simulink model "c6_formation"  (R2021b)
settings: Solver=FixedStepDiscrete  StartTime=0.0  StopTime=Inf  FixedStep=sampleTime  RelTol=1e-3  EnableMultiTasking=on
PreLoadFcn:
  | %load emptyMap
  | 
  | % Lidar parameters
  | sensorOffset = [0,0];
  | scanAngles = -pi:pi/6:pi;
  | maxRange = 0.25;
InitFcn:
  | sampleTime = 0.05;
  | nMedianSize=3;
  | 
  | % Robot parameters
  | wheelRadius = 0.0335;
  | robotRadius = 0.116/2;
  | 
  | %角速度坐标
  | ks=1;
  | 
  | % Lidar parameters
  | sensorOffset = [0,0];
  | scanAngles = -pi/3:pi/36:pi/3;
  | maxRange = 0.2;
  | 
  | %车初始位置
  | init_pose_1=[1  1.3  pi/2]';
  | init_pose_2=[0.85 1  pi/2]';
  | init_pose_3=[1.15 1  pi/2]';
  | init_pose_4=[0.7  0.7 pi/2]';
  | init_pose_5=[1  0.7 pi/2]';
  | init_pose_6=[1.3 0.7  pi/2]';
  | 
  | %pp算法性能参数
  | Vd_pp=0.2;
  | Wd_pp=pi;
  | dist_pp=0.2;
  | GoalRadius=0.1;
  | numSector=180;
  | rangeDis=[0.1,maxRange];
  | thresholds=[1/360 1/36];
  | safetyDis=0.2;
  | minimumTurningRadius=0.5*robotRadius;
  | recovery_w=0.05;
undefined symbols (not defined in the file): Angular, DiscIntNeverNeededParam, Linear
libraries: robotlib x24, dspstat3 x18, robotalgslib x6
(part 3 of 4)

== system c6_formation/controller/Car5/ppCar/Adjust Velocities to Avoid Obstacles/Path Following ==
  SteeringDirection : Inport
  V : Inport  Port=2
  AngularVelocity : Inport  Port=3
  Action Port : ActionPort
  Compute Angular Velocity : MATLAB Function  TreatAsAtomicUnit=on
  Constant : Constant  Value=0
  Gain : Gain  Gain=0.2
  MaxAngularVelocity : Constant
  Subtract : Sum  Inputs=+-
  Subtract1 : Sum  Inputs=+-
  dV : Outport  VectorParamsAs1DForOutWhenUnconnected=off
  dW : Outport  Port=2  VectorParamsAs1DForOutWhenUnconnected=off
  wires:
  AngularVelocity/1 -> Subtract/2
  Compute Angular Velocity/1(w) -> Subtract/1
  Subtract/1 -> dW/1
  SteeringDirection/1 -> Compute Angular Velocity/1(steeringDir)
  MaxAngularVelocity/1 -> Compute Angular Velocity/2(wMax)
  Subtract1/1 -> dV/1
  V/1 -> Gain/1
  Constant/1 -> Subtract1/1
  Gain/1 -> Subtract1/2

== system c6_formation/controller/Car5/ppCar/Adjust Velocities to Avoid Obstacles/Recovery ==
  LinearVelocity : Inport
  AngularVelocity : Inport  Port=2
  Action Port : ActionPort
  Constant1 : Constant  Value=-pi/2
  Constant2 : Constant  Value=recovery_w
  Gain : Gain  Gain=-1
  Subtract : Sum  Inputs=+-
  Subtract1 : Sum  Inputs=+-
  dV : Outport  VectorParamsAs1DForOutWhenUnconnected=off
  dW : Outport  Port=2  VectorParamsAs1DForOutWhenUnconnected=off
  wires:
  Subtract/1 -> dW/1
  AngularVelocity/1 -> Subtract/2
  Subtract1/1 -> dV/1
  LinearVelocity/1 -> Gain/1
  Gain/1 -> Subtract1/1
  Constant2/1 -> Subtract1/2
  Constant1/1 -> Subtract/1

== system c6_formation/controller/Car5/ppCar/Compute Velocity and Heading for Path following/Car1 ==
  pose : Inport
  waypoint : Inport  Port=2
  Demux : Demux  Outputs=3
  Demux1 : Demux  Outputs=3
  Ground : Ground
  Kinematicc Controller : Subsystem  mask(Kinematic Controller){kx=2, ky=2, lx=2, ly=2, kw=3, lw=3, Vmax=0.3, Wmax=pi}
      mask prompts: kx "横向偏差增益: kx"; ky "纵向偏差增益: ky"; lx "横向输出饱和: lx"; ly "纵向输出饱和: ly"; kw "离心线速度转角速度增益"; lw "离心线速度转角速度增益"; Vmax "车的限制速度"; Wmax "车的限制角速度"
      mask help: This block implements a controller for differential-drive mobile robots to follow a desired trajectory or to go to a goal point.
      mask Help:
      | This block implements a controller for differential-drive mobile robots to follow a desired trajectory or to go to a goal point.
      | 
      | The trajectory tracking controller is based on the inverse kinematics of the differential-drive robot, whereas only the position [x, y] of the point of interest is considered.
      | It generates references for linear and angular velocities [ud, wd] based on the robot's actual pose [x, y, psi] deseired position [xd, yd] and desired speed [dxd, dyd].
      | 
      | The constant "a" represents the distance of the point of interest [x, y] to the center of the line that connects the traction wheels.
      | 
      | <b>Parameters:</b>
      | 
      | kx > 0 and ky > 0: controller gains;
      | lx > 0 and ly > 0: saturation constants.
      | 
      | 
      | <b>Inputs:</b>
      | 
      | psi: actual robot orientation [rad] (psi=0 means the robot orientation is the same as the x axis);
      | x: actual robot position [m] in x axis;
      | xd: desired robot position [m] in x axis;
      | dxd: desired robot speed [m/s] in x axis;
      | y: actual robot position [m] in y axis;
      | yd: desired robot position [m] in y axis;
      | dyd: desired robot speed [m/s] in y axis;
      | 
      | <b>Outputs:</b>
      | 
      | ud: reference for linear velocity [m/s]
      | wd: reference for angular velocity [rad/s]
      | 
      | 
      | <b>Notes:</b>
      | 
      | If the deseired position [xd, yd] is constant and the desired speed [dxd, dyd] is zero, the controller works as a position controller: it drives the robot to a goal position [xd, yd].
      | 
      | ------
      | For detailed information on the system, please refer to the following papers and thesis:
      | 
      | [1] MARTINS, F. N., Celeste, W. C., Carelli, R., Sarcinelli-Filho, M. and
      | Bastos-Filho, T. F. An Adaptive Dynamic Controller for Autonomous Mobile Robot
      | Trajectory Tracking. Control Engineering Practice, v. 16, p. 1354–1363, 2008.
      | doi: 10.1016/j.conengprac.2008.03.004
      | 
      | [2] MARTINS, F. N., Carelli, R., Sarcinelli-Filho, M. and Bastos-Filho, T. F.
      | Dynamic Modeling and Adaptive Dynamic Compensation for Unicycle-Like
      | Mobile Robots. 14th International Conference on Advanced Robotics -
      | ICAR 2009, Germany, June, 22-26, 2009.
      | 
      | [3] Thesis: "Modelagem e Compensacao da Dinamica de Robos Moveis e sua
      | Aplicacao em Controle de Formacao". Felipe Nascimento Martins. Tese de
      | Doutorado em Engenharia Eletrica - Automacao. UFES, 2009.
      | 
      | ---
      | Based on a prior work by Felipe Nascimento Martins and Wanderley Cardoso Celeste
      | UFES - Federal University of Espirito Santo, BRAZIL
      | 2006--2008
      | 
      | Author: Felipe Nascimento Martins
      | Federal Institute of Education, Science and Technology of Espirito Santo - IFES
      | NERA - Núcleo de Estudos em Robótica e Automação
      | http://nera.sr.ifes.edu.br
      | MAY/2013
      | Blog sobre robótica: www.nossosrobos.blogspot.com
  V : Outport
  W : Outport  Port=2
  targetdir : Outport  Port=3
  wires:
  Ground/1 -> Kinematicc Controller/7(dxd), Kinematicc Controller/8(dyd)
  Demux1/2 -> Kinematicc Controller/5(yd)
  Kinematicc Controller/1(ud) -> V/1  "速度指令"
  Demux/2 -> Kinematicc Controller/2(y)
  pose/1 -> Demux/1
  Demux/3 -> Kinematicc Controller/3(psi)
  Demux/1 -> Kinematicc Controller/1(x)
  Kinematicc Controller/2(wd) -> W/1  "角速度指令"
  Demux1/1 -> Kinematicc Controller/4(xd)
  waypoint/1 -> Demux1/1
  Demux1/3 -> Kinematicc Controller/6(psid)
  Kinematicc Controller/3(targetdir) -> targetdir/1

== system c6_formation/controller/Car6/ppCar/Adjust Velocities to Avoid Obstacles/Path Following ==
  SteeringDirection : Inport
  V : Inport  Port=2
  AngularVelocity : Inport  Port=3
  Action Port : ActionPort
  Compute Angular Velocity : MATLAB Function  TreatAsAtomicUnit=on
  Constant : Constant  Value=0
  Gain : Gain  Gain=0.2
  MaxAngularVelocity : Constant
  Subtract : Sum  Inputs=+-
  Subtract1 : Sum  Inputs=+-
  dV : Outport  VectorParamsAs1DForOutWhenUnconnected=off
  dW : Outport  Port=2  VectorParamsAs1DForOutWhenUnconnected=off
  wires:
  Gain/1 -> Subtract1/2
  Constant/1 -> Subtract1/1
  V/1 -> Gain/1
  Subtract1/1 -> dV/1
  MaxAngularVelocity/1 -> Compute Angular Velocity/2(wMax)
  SteeringDirection/1 -> Compute Angular Velocity/1(steeringDir)
  Subtract/1 -> dW/1
  Compute Angular Velocity/1(w) -> Subtract/1
  AngularVelocity/1 -> Subtract/2

== system c6_formation/controller/Car6/ppCar/Adjust Velocities to Avoid Obstacles/Recovery ==
  LinearVelocity : Inport
  AngularVelocity : Inport  Port=2
  Action Port : ActionPort
  Constant1 : Constant  Value=-pi/2
  Constant2 : Constant  Value=recovery_w
  Gain : Gain  Gain=-1
  Subtract : Sum  Inputs=+-
  Subtract1 : Sum  Inputs=+-
  dV : Outport  VectorParamsAs1DForOutWhenUnconnected=off
  dW : Outport  Port=2  VectorParamsAs1DForOutWhenUnconnected=off
  wires:
  Constant1/1 -> Subtract/1
  Constant2/1 -> Subtract1/2
  Gain/1 -> Subtract1/1
  LinearVelocity/1 -> Gain/1
  Subtract1/1 -> dV/1
  AngularVelocity/1 -> Subtract/2
  Subtract/1 -> dW/1

== system c6_formation/controller/Car6/ppCar/Compute Velocity and Heading for Path following/Car1 ==
  pose : Inport
  waypoint : Inport  Port=2
  Demux : Demux  Outputs=3
  Demux1 : Demux  Outputs=3
  Ground : Ground
  Kinematicc Controller : Subsystem  mask(Kinematic Controller){kx=2, ky=2, lx=2, ly=2, kw=3, lw=3, Vmax=0.3, Wmax=pi}
      mask prompts: kx "横向偏差增益: kx"; ky "纵向偏差增益: ky"; lx "横向输出饱和: lx"; ly "纵向输出饱和: ly"; kw "离心线速度转角速度增益"; lw "离心线速度转角速度增益"; Vmax "车的限制速度"; Wmax "车的限制角速度"
      mask help: This block implements a controller for differential-drive mobile robots to follow a desired trajectory or to go to a goal point.
      mask Help:
      | This block implements a controller for differential-drive mobile robots to follow a desired trajectory or to go to a goal point.
      | 
      | The trajectory tracking controller is based on the inverse kinematics of the differential-drive robot, whereas only the position [x, y] of the point of interest is considered.
      | It generates references for linear and angular velocities [ud, wd] based on the robot's actual pose [x, y, psi] deseired position [xd, yd] and desired speed [dxd, dyd].
      | 
      | The constant "a" represents the distance of the point of interest [x, y] to the center of the line that connects the traction wheels.
      | 
      | <b>Parameters:</b>
      | 
      | kx > 0 and ky > 0: controller gains;
      | lx > 0 and ly > 0: saturation constants.
      | 
      | 
      | <b>Inputs:</b>
      | 
      | psi: actual robot orientation [rad] (psi=0 means the robot orientation is the same as the x axis);
      | x: actual robot position [m] in x axis;
      | xd: desired robot position [m] in x axis;
      | dxd: desired robot speed [m/s] in x axis;
      | y: actual robot position [m] in y axis;
      | yd: desired robot position [m] in y axis;
      | dyd: desired robot speed [m/s] in y axis;
      | 
      | <b>Outputs:</b>
      | 
      | ud: reference for linear velocity [m/s]
      | wd: reference for angular velocity [rad/s]
      | 
      | 
      | <b>Notes:</b>
      | 
      | If the deseired position [xd, yd] is constant and the desired speed [dxd, dyd] is zero, the controller works as a position controller: it drives the robot to a goal position [xd, yd].
      | 
      | ------
      | For detailed information on the system, please refer to the following papers and thesis:
      | 
      | [1] MARTINS, F. N., Celeste, W. C., Carelli, R., Sarcinelli-Filho, M. and
      | Bastos-Filho, T. F. An Adaptive Dynamic Controller for Autonomous Mobile Robot
      | Trajectory Tracking. Control Engineering Practice, v. 16, p. 1354–1363, 2008.
      | doi: 10.1016/j.conengprac.2008.03.004
      | 
      | [2] MARTINS, F. N., Carelli, R., Sarcinelli-Filho, M. and Bastos-Filho, T. F.
      | Dynamic Modeling and Adaptive Dynamic Compensation for Unicycle-Like
      | Mobile Robots. 14th International Conference on Advanced Robotics -
      | ICAR 2009, Germany, June, 22-26, 2009.
      | 
      | [3] Thesis: "Modelagem e Compensacao da Dinamica de Robos Moveis e sua
      | Aplicacao em Controle de Formacao". Felipe Nascimento Martins. Tese de
      | Doutorado em Engenharia Eletrica - Automacao. UFES, 2009.
      | 
      | ---
      | Based on a prior work by Felipe Nascimento Martins and Wanderley Cardoso Celeste
      | UFES - Federal University of Espirito Santo, BRAZIL
      | 2006--2008
      | 
      | Author: Felipe Nascimento Martins
      | Federal Institute of Education, Science and Technology of Espirito Santo - IFES
      | NERA - Núcleo de Estudos em Robótica e Automação
      | http://nera.sr.ifes.edu.br
      | MAY/2013
      | Blog sobre robótica: www.nossosrobos.blogspot.com
  V : Outport
  W : Outport  Port=2
  targetdir : Outport  Port=3
  wires:
  Kinematicc Controller/3(targetdir) -> targetdir/1
  Demux1/3 -> Kinematicc Controller/6(psid)
  waypoint/1 -> Demux1/1
  Demux1/1 -> Kinematicc Controller/4(xd)
  Kinematicc Controller/2(wd) -> W/1  "角速度指令"
  Demux/1 -> Kinematicc Controller/1(x)
  Demux/3 -> Kinematicc Controller/3(psi)
  pose/1 -> Demux/1
  Demux/2 -> Kinematicc Controller/2(y)
  Kinematicc Controller/1(ud) -> V/1  "速度指令"
  Demux1/2 -> Kinematicc Controller/5(yd)
  Ground/1 -> Kinematicc Controller/8(dyd), Kinematicc Controller/7(dxd)

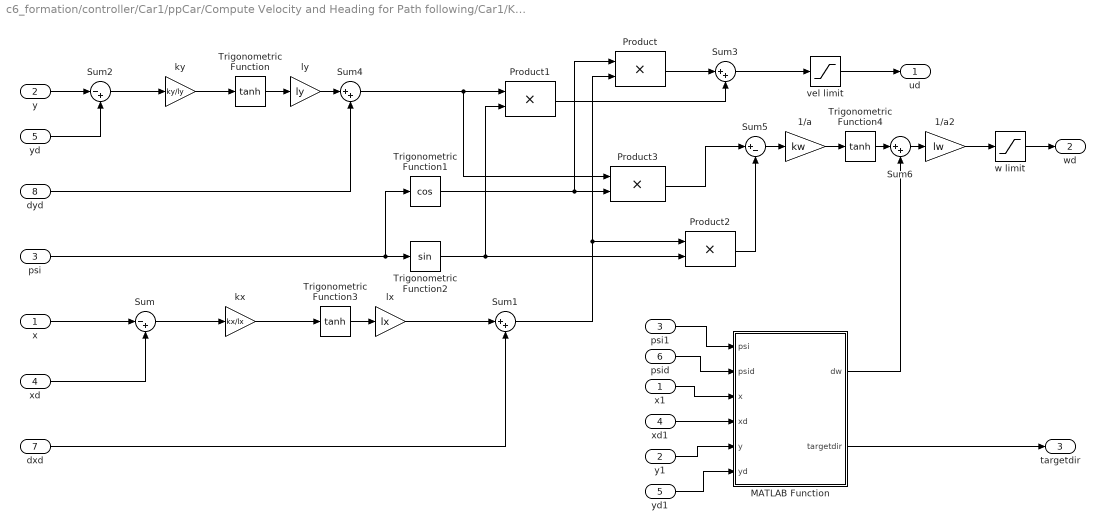
== system c6_formation/controller/Car1/ppCar/Compute Velocity and Heading for Path following/Car1/Kinematicc Controller ==
  x : Inport
  y : Inport  Port=2
  psi : Inport  Port=3
  xd : Inport  Port=4
  yd : Inport  Port=5
  psid : Inport  Port=6
  dxd : Inport  Port=7
  dyd : Inport  Port=8
  1/a : Gain  Gain=kw  SaturateOnIntegerOverflow=on  OutDataTypeStr=Inherit: Same as input  ParamDataTypeStr=Inherit: Same as input
  1/a2 : Gain  Gain=lw  SaturateOnIntegerOverflow=on  OutDataTypeStr=Inherit: Same as input  ParamDataTypeStr=Inherit: Same as input
  MATLAB Function : MATLAB Function  TreatAsAtomicUnit=on
  Product{,1..3} (4 alike) : Product  SaturateOnIntegerOverflow=on  OutDataTypeStr=Inherit: Same as first input
  Sum : Sum  Inputs=|-+  SaturateOnIntegerOverflow=on
  Sum{1,3..4,6} (4 alike) : Sum  Inputs=|++  SaturateOnIntegerOverflow=on
  Sum2 : Sum  Inputs=|-+  SaturateOnIntegerOverflow=on
  Sum5 : Sum  Inputs=|+-  SaturateOnIntegerOverflow=on
  Trigonometric Function : Trigonometry  Operator=tanh
  Trigonometric Function1 : Trigonometry  Operator=cos
  Trigonometric Function2 : Trigonometry
  Trigonometric Function3 : Trigonometry  Operator=tanh
  Trigonometric Function4 : Trigonometry  Operator=tanh
  kx : Gain  Gain=kx/lx  SaturateOnIntegerOverflow=on  OutDataTypeStr=Inherit: Same as input  ParamDataTypeStr=Inherit: Same as input
  ky : Gain  Gain=ky/ly  SaturateOnIntegerOverflow=on  OutDataTypeStr=Inherit: Same as input  ParamDataTypeStr=Inherit: Same as input
  lx : Gain  Gain=lx  SaturateOnIntegerOverflow=on  OutDataTypeStr=Inherit: Same as input  ParamDataTypeStr=Inherit: Same as input
  ly : Gain  Gain=ly  SaturateOnIntegerOverflow=on  OutDataTypeStr=Inherit: Same as input  ParamDataTypeStr=Inherit: Same as input
  psi1 : InportShadow  Port=3
  vel limit : Saturate  UpperLimit=Vmax  LowerLimit=-0.4*Vmax
  w limit : Saturate  UpperLimit=Wmax  LowerLimit=-Wmax
  x1 : InportShadow
  xd1 : InportShadow  Port=4
  y1 : InportShadow  Port=2
  yd1 : InportShadow  Port=5
  ud : Outport
  wd : Outport  Port=2
  targetdir : Outport  Port=3
  wires:
  kx/1 -> Trigonometric Function3/1
  ky/1 -> Trigonometric Function/1
  Trigonometric Function1/1 -> Product3/2, Product/1
  Sum/1 -> kx/1
  y/1 -> Sum2/1
  Sum4/1 -> Product1/1, Product3/1
  Trigonometric Function2/1 -> Product2/2, Product1/2
  Sum3/1 -> vel limit/1
  dxd/1 -> Sum1/2
  dyd/1 -> Sum4/2
  ly/1 -> Sum4/1
  Trigonometric Function/1 -> ly/1
  lx/1 -> Sum1/1
  Trigonometric Function3/1 -> lx/1
  yd/1 -> Sum2/2
  xd/1 -> Sum/2
  x/1 -> Sum/1
  psi/1 -> Trigonometric Function2/1, Trigonometric Function1/1
  Sum1/1 -> Product2/1, Product/2
  Sum2/1 -> ky/1
  Product/1 -> Sum3/1
  Product1/1 -> Sum3/2
  Product3/1 -> Sum5/1
  Product2/1 -> Sum5/2
  Sum5/1 -> 1/a/1
  Trigonometric Function4/1 -> Sum6/1
  1/a/1 -> Trigonometric Function4/1
  vel limit/1 -> ud/1
  w limit/1 -> wd/1
  1/a2/1 -> w limit/1
  Sum6/1 -> 1/a2/1
  psid/1 -> MATLAB Function/2(psid)
  psi1/1 -> MATLAB Function/1(psi)
  x1/1 -> MATLAB Function/3(x)
  xd1/1 -> MATLAB Function/4(xd)
  y1/1 -> MATLAB Function/5(y)
  yd1/1 -> MATLAB Function/6(yd)
  MATLAB Function/1(dw) -> Sum6/2
  MATLAB Function/2(targetdir) -> targetdir/1

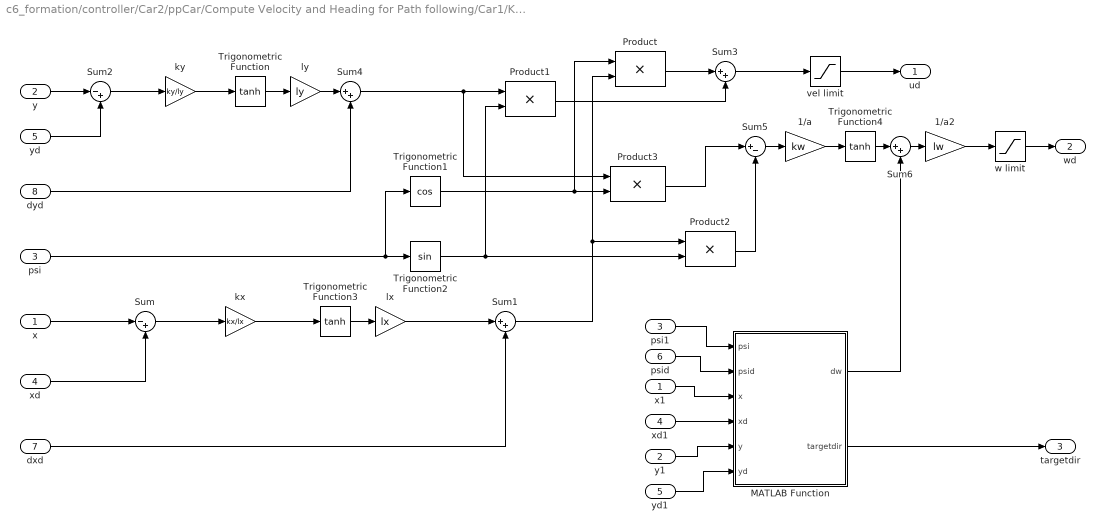
== system c6_formation/controller/Car2/ppCar/Compute Velocity and Heading for Path following/Car1/Kinematicc Controller ==
  x : Inport
  y : Inport  Port=2
  psi : Inport  Port=3
  xd : Inport  Port=4
  yd : Inport  Port=5
  psid : Inport  Port=6
  dxd : Inport  Port=7
  dyd : Inport  Port=8
  1/a : Gain  Gain=kw  SaturateOnIntegerOverflow=on  OutDataTypeStr=Inherit: Same as input  ParamDataTypeStr=Inherit: Same as input
  1/a2 : Gain  Gain=lw  SaturateOnIntegerOverflow=on  OutDataTypeStr=Inherit: Same as input  ParamDataTypeStr=Inherit: Same as input
  MATLAB Function : MATLAB Function  TreatAsAtomicUnit=on
  Product{,1..3} (4 alike) : Product  SaturateOnIntegerOverflow=on  OutDataTypeStr=Inherit: Same as first input
  Sum : Sum  Inputs=|-+  SaturateOnIntegerOverflow=on
  Sum{1,3..4,6} (4 alike) : Sum  Inputs=|++  SaturateOnIntegerOverflow=on
  Sum2 : Sum  Inputs=|-+  SaturateOnIntegerOverflow=on
  Sum5 : Sum  Inputs=|+-  SaturateOnIntegerOverflow=on
  Trigonometric Function : Trigonometry  Operator=tanh
  Trigonometric Function1 : Trigonometry  Operator=cos
  Trigonometric Function2 : Trigonometry
  Trigonometric Function3 : Trigonometry  Operator=tanh
  Trigonometric Function4 : Trigonometry  Operator=tanh
  kx : Gain  Gain=kx/lx  SaturateOnIntegerOverflow=on  OutDataTypeStr=Inherit: Same as input  ParamDataTypeStr=Inherit: Same as input
  ky : Gain  Gain=ky/ly  SaturateOnIntegerOverflow=on  OutDataTypeStr=Inherit: Same as input  ParamDataTypeStr=Inherit: Same as input
  lx : Gain  Gain=lx  SaturateOnIntegerOverflow=on  OutDataTypeStr=Inherit: Same as input  ParamDataTypeStr=Inherit: Same as input
  ly : Gain  Gain=ly  SaturateOnIntegerOverflow=on  OutDataTypeStr=Inherit: Same as input  ParamDataTypeStr=Inherit: Same as input
  psi1 : InportShadow  Port=3
  vel limit : Saturate  UpperLimit=Vmax  LowerLimit=-0.4*Vmax
  w limit : Saturate  UpperLimit=Wmax  LowerLimit=-Wmax
  x1 : InportShadow
  xd1 : InportShadow  Port=4
  y1 : InportShadow  Port=2
  yd1 : InportShadow  Port=5
  ud : Outport
  wd : Outport  Port=2
  targetdir : Outport  Port=3
  wires:
  MATLAB Function/2(targetdir) -> targetdir/1
  MATLAB Function/1(dw) -> Sum6/2
  yd1/1 -> MATLAB Function/6(yd)
  y1/1 -> MATLAB Function/5(y)
  xd1/1 -> MATLAB Function/4(xd)
  x1/1 -> MATLAB Function/3(x)
  psi1/1 -> MATLAB Function/1(psi)
  psid/1 -> MATLAB Function/2(psid)
  Sum6/1 -> 1/a2/1
  1/a2/1 -> w limit/1
  w limit/1 -> wd/1
  vel limit/1 -> ud/1
  1/a/1 -> Trigonometric Function4/1
  Trigonometric Function4/1 -> Sum6/1
  Sum5/1 -> 1/a/1
  Product2/1 -> Sum5/2
  Product3/1 -> Sum5/1
  Product1/1 -> Sum3/2
  Product/1 -> Sum3/1
  Sum2/1 -> ky/1
  Sum1/1 -> Product/2, Product2/1
  psi/1 -> Trigonometric Function1/1, Trigonometric Function2/1
  x/1 -> Sum/1
  xd/1 -> Sum/2
  yd/1 -> Sum2/2
  Trigonometric Function3/1 -> lx/1
  lx/1 -> Sum1/1
  Trigonometric Function/1 -> ly/1
  ly/1 -> Sum4/1
  dyd/1 -> Sum4/2
  dxd/1 -> Sum1/2
  Sum3/1 -> vel limit/1
  Trigonometric Function2/1 -> Product1/2, Product2/2
  Sum4/1 -> Product3/1, Product1/1
  y/1 -> Sum2/1
  Sum/1 -> kx/1
  Trigonometric Function1/1 -> Product/1, Product3/2
  ky/1 -> Trigonometric Function/1
  kx/1 -> Trigonometric Function3/1

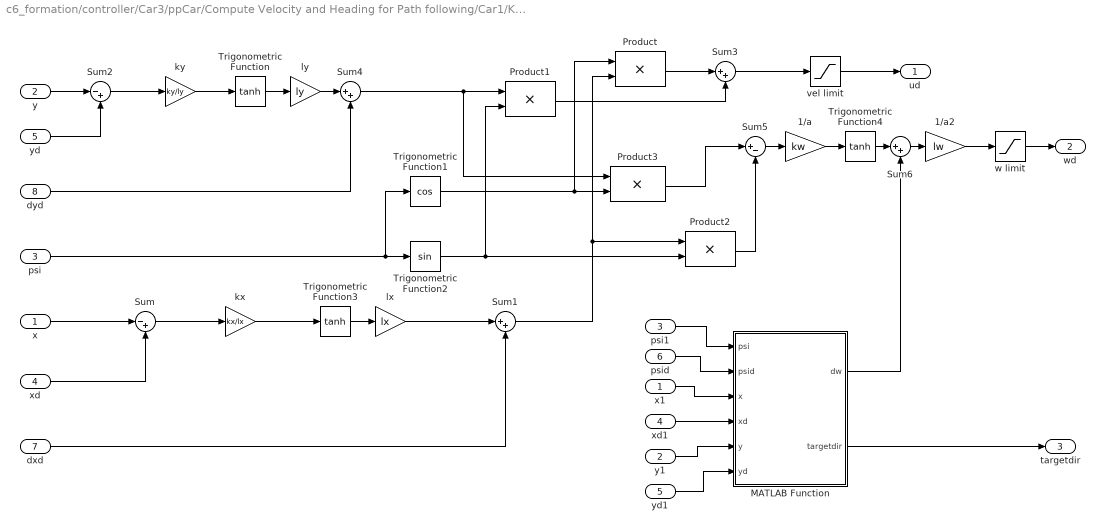
== system c6_formation/controller/Car3/ppCar/Compute Velocity and Heading for Path following/Car1/Kinematicc Controller ==
  x : Inport
  y : Inport  Port=2
  psi : Inport  Port=3
  xd : Inport  Port=4
  yd : Inport  Port=5
  psid : Inport  Port=6
  dxd : Inport  Port=7
  dyd : Inport  Port=8
  1/a : Gain  Gain=kw  SaturateOnIntegerOverflow=on  OutDataTypeStr=Inherit: Same as input  ParamDataTypeStr=Inherit: Same as input
  1/a2 : Gain  Gain=lw  SaturateOnIntegerOverflow=on  OutDataTypeStr=Inherit: Same as input  ParamDataTypeStr=Inherit: Same as input
  MATLAB Function : MATLAB Function  TreatAsAtomicUnit=on
  Product{,1..3} (4 alike) : Product  SaturateOnIntegerOverflow=on  OutDataTypeStr=Inherit: Same as first input
  Sum : Sum  Inputs=|-+  SaturateOnIntegerOverflow=on
  Sum{1,3..4,6} (4 alike) : Sum  Inputs=|++  SaturateOnIntegerOverflow=on
  Sum2 : Sum  Inputs=|-+  SaturateOnIntegerOverflow=on
  Sum5 : Sum  Inputs=|+-  SaturateOnIntegerOverflow=on
  Trigonometric Function : Trigonometry  Operator=tanh
  Trigonometric Function1 : Trigonometry  Operator=cos
  Trigonometric Function2 : Trigonometry
  Trigonometric Function3 : Trigonometry  Operator=tanh
  Trigonometric Function4 : Trigonometry  Operator=tanh
  kx : Gain  Gain=kx/lx  SaturateOnIntegerOverflow=on  OutDataTypeStr=Inherit: Same as input  ParamDataTypeStr=Inherit: Same as input
  ky : Gain  Gain=ky/ly  SaturateOnIntegerOverflow=on  OutDataTypeStr=Inherit: Same as input  ParamDataTypeStr=Inherit: Same as input
  lx : Gain  Gain=lx  SaturateOnIntegerOverflow=on  OutDataTypeStr=Inherit: Same as input  ParamDataTypeStr=Inherit: Same as input
  ly : Gain  Gain=ly  SaturateOnIntegerOverflow=on  OutDataTypeStr=Inherit: Same as input  ParamDataTypeStr=Inherit: Same as input
  psi1 : InportShadow  Port=3
  vel limit : Saturate  UpperLimit=Vmax  LowerLimit=-0.4*Vmax
  w limit : Saturate  UpperLimit=Wmax  LowerLimit=-Wmax
  x1 : InportShadow
  xd1 : InportShadow  Port=4
  y1 : InportShadow  Port=2
  yd1 : InportShadow  Port=5
  ud : Outport
  wd : Outport  Port=2
  targetdir : Outport  Port=3
  wires:
  kx/1 -> Trigonometric Function3/1
  ky/1 -> Trigonometric Function/1
  Trigonometric Function1/1 -> Product3/2, Product/1
  Sum/1 -> kx/1
  y/1 -> Sum2/1
  Sum4/1 -> Product1/1, Product3/1
  Trigonometric Function2/1 -> Product2/2, Product1/2
  Sum3/1 -> vel limit/1
  dxd/1 -> Sum1/2
  dyd/1 -> Sum4/2
  ly/1 -> Sum4/1
  Trigonometric Function/1 -> ly/1
  lx/1 -> Sum1/1
  Trigonometric Function3/1 -> lx/1
  yd/1 -> Sum2/2
  xd/1 -> Sum/2
  x/1 -> Sum/1
  psi/1 -> Trigonometric Function2/1, Trigonometric Function1/1
  Sum1/1 -> Product2/1, Product/2
  Sum2/1 -> ky/1
  Product/1 -> Sum3/1
  Product1/1 -> Sum3/2
  Product3/1 -> Sum5/1
  Product2/1 -> Sum5/2
  Sum5/1 -> 1/a/1
  Trigonometric Function4/1 -> Sum6/1
  1/a/1 -> Trigonometric Function4/1
  vel limit/1 -> ud/1
  w limit/1 -> wd/1
  1/a2/1 -> w limit/1
  Sum6/1 -> 1/a2/1
  psid/1 -> MATLAB Function/2(psid)
  psi1/1 -> MATLAB Function/1(psi)
  x1/1 -> MATLAB Function/3(x)
  xd1/1 -> MATLAB Function/4(xd)
  y1/1 -> MATLAB Function/5(y)
  yd1/1 -> MATLAB Function/6(yd)
  MATLAB Function/1(dw) -> Sum6/2
  MATLAB Function/2(targetdir) -> targetdir/1

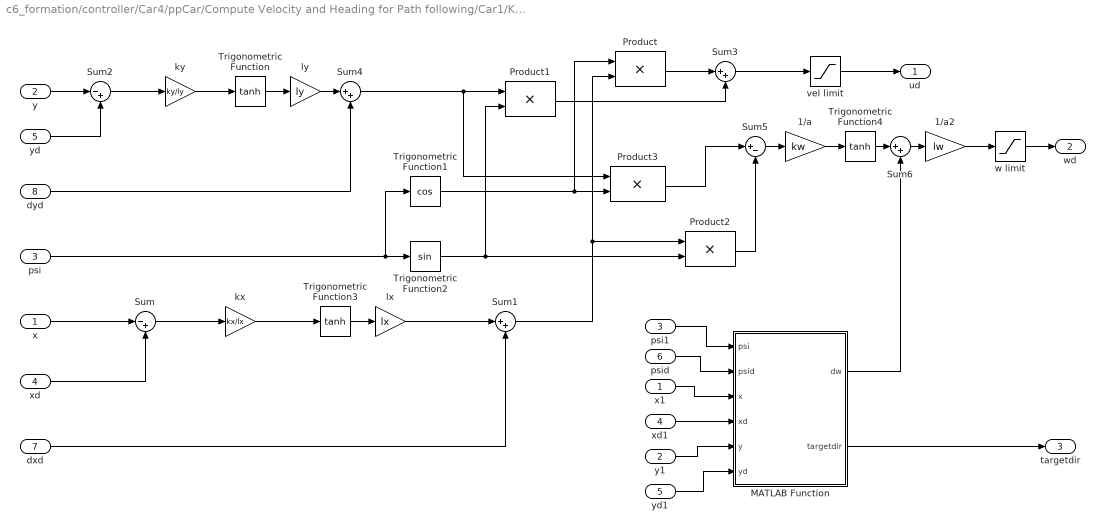
== system c6_formation/controller/Car4/ppCar/Compute Velocity and Heading for Path following/Car1/Kinematicc Controller ==
  x : Inport
  y : Inport  Port=2
  psi : Inport  Port=3
  xd : Inport  Port=4
  yd : Inport  Port=5
  psid : Inport  Port=6
  dxd : Inport  Port=7
  dyd : Inport  Port=8
  1/a : Gain  Gain=kw  SaturateOnIntegerOverflow=on  OutDataTypeStr=Inherit: Same as input  ParamDataTypeStr=Inherit: Same as input
  1/a2 : Gain  Gain=lw  SaturateOnIntegerOverflow=on  OutDataTypeStr=Inherit: Same as input  ParamDataTypeStr=Inherit: Same as input
  MATLAB Function : MATLAB Function  TreatAsAtomicUnit=on
  Product{,1..3} (4 alike) : Product  SaturateOnIntegerOverflow=on  OutDataTypeStr=Inherit: Same as first input
  Sum : Sum  Inputs=|-+  SaturateOnIntegerOverflow=on
  Sum{1,3..4,6} (4 alike) : Sum  Inputs=|++  SaturateOnIntegerOverflow=on
  Sum2 : Sum  Inputs=|-+  SaturateOnIntegerOverflow=on
  Sum5 : Sum  Inputs=|+-  SaturateOnIntegerOverflow=on
  Trigonometric Function : Trigonometry  Operator=tanh
  Trigonometric Function1 : Trigonometry  Operator=cos
  Trigonometric Function2 : Trigonometry
  Trigonometric Function3 : Trigonometry  Operator=tanh
  Trigonometric Function4 : Trigonometry  Operator=tanh
  kx : Gain  Gain=kx/lx  SaturateOnIntegerOverflow=on  OutDataTypeStr=Inherit: Same as input  ParamDataTypeStr=Inherit: Same as input
  ky : Gain  Gain=ky/ly  SaturateOnIntegerOverflow=on  OutDataTypeStr=Inherit: Same as input  ParamDataTypeStr=Inherit: Same as input
  lx : Gain  Gain=lx  SaturateOnIntegerOverflow=on  OutDataTypeStr=Inherit: Same as input  ParamDataTypeStr=Inherit: Same as input
  ly : Gain  Gain=ly  SaturateOnIntegerOverflow=on  OutDataTypeStr=Inherit: Same as input  ParamDataTypeStr=Inherit: Same as input
  psi1 : InportShadow  Port=3
  vel limit : Saturate  UpperLimit=Vmax  LowerLimit=-0.4*Vmax
  w limit : Saturate  UpperLimit=Wmax  LowerLimit=-Wmax
  x1 : InportShadow
  xd1 : InportShadow  Port=4
  y1 : InportShadow  Port=2
  yd1 : InportShadow  Port=5
  ud : Outport
  wd : Outport  Port=2
  targetdir : Outport  Port=3
  wires:
  MATLAB Function/2(targetdir) -> targetdir/1
  MATLAB Function/1(dw) -> Sum6/2
  yd1/1 -> MATLAB Function/6(yd)
  y1/1 -> MATLAB Function/5(y)
  xd1/1 -> MATLAB Function/4(xd)
  x1/1 -> MATLAB Function/3(x)
  psi1/1 -> MATLAB Function/1(psi)
  psid/1 -> MATLAB Function/2(psid)
  Sum6/1 -> 1/a2/1
  1/a2/1 -> w limit/1
  w limit/1 -> wd/1
  vel limit/1 -> ud/1
  1/a/1 -> Trigonometric Function4/1
  Trigonometric Function4/1 -> Sum6/1
  Sum5/1 -> 1/a/1
  Product2/1 -> Sum5/2
  Product3/1 -> Sum5/1
  Product1/1 -> Sum3/2
  Product/1 -> Sum3/1
  Sum2/1 -> ky/1
  Sum1/1 -> Product/2, Product2/1
  psi/1 -> Trigonometric Function1/1, Trigonometric Function2/1
  x/1 -> Sum/1
  xd/1 -> Sum/2
  yd/1 -> Sum2/2
  Trigonometric Function3/1 -> lx/1
  lx/1 -> Sum1/1
  Trigonometric Function/1 -> ly/1
  ly/1 -> Sum4/1
  dyd/1 -> Sum4/2
  dxd/1 -> Sum1/2
  Sum3/1 -> vel limit/1
  Trigonometric Function2/1 -> Product1/2, Product2/2
  Sum4/1 -> Product3/1, Product1/1
  y/1 -> Sum2/1
  Sum/1 -> kx/1
  Trigonometric Function1/1 -> Product/1, Product3/2
  ky/1 -> Trigonometric Function/1
  kx/1 -> Trigonometric Function3/1

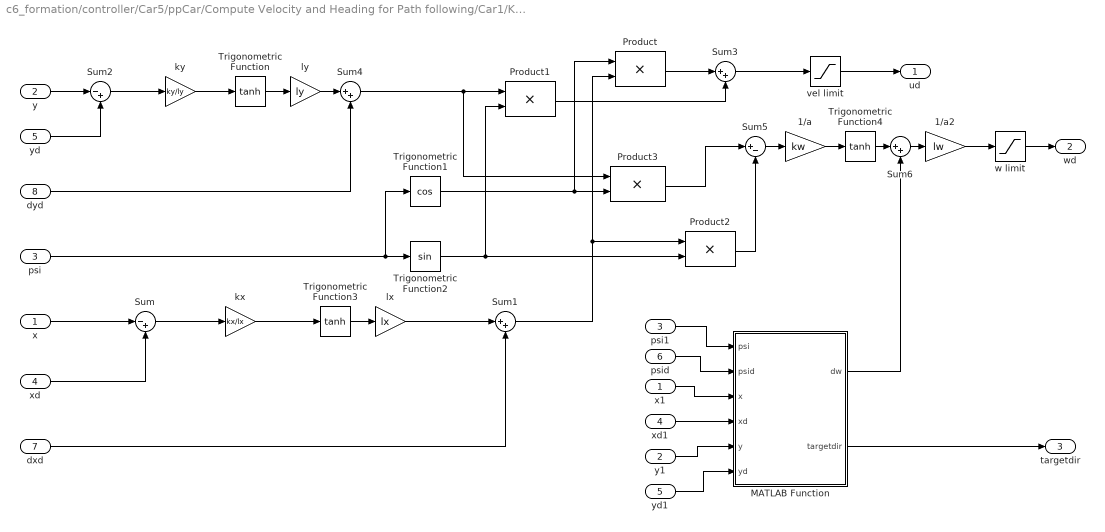
== system c6_formation/controller/Car5/ppCar/Compute Velocity and Heading for Path following/Car1/Kinematicc Controller ==
  x : Inport
  y : Inport  Port=2
  psi : Inport  Port=3
  xd : Inport  Port=4
  yd : Inport  Port=5
  psid : Inport  Port=6
  dxd : Inport  Port=7
  dyd : Inport  Port=8
  1/a : Gain  Gain=kw  SaturateOnIntegerOverflow=on  OutDataTypeStr=Inherit: Same as input  ParamDataTypeStr=Inherit: Same as input
  1/a2 : Gain  Gain=lw  SaturateOnIntegerOverflow=on  OutDataTypeStr=Inherit: Same as input  ParamDataTypeStr=Inherit: Same as input
  MATLAB Function : MATLAB Function  TreatAsAtomicUnit=on
  Product{,1..3} (4 alike) : Product  SaturateOnIntegerOverflow=on  OutDataTypeStr=Inherit: Same as first input
  Sum : Sum  Inputs=|-+  SaturateOnIntegerOverflow=on
  Sum{1,3..4,6} (4 alike) : Sum  Inputs=|++  SaturateOnIntegerOverflow=on
  Sum2 : Sum  Inputs=|-+  SaturateOnIntegerOverflow=on
  Sum5 : Sum  Inputs=|+-  SaturateOnIntegerOverflow=on
  Trigonometric Function : Trigonometry  Operator=tanh
  Trigonometric Function1 : Trigonometry  Operator=cos
  Trigonometric Function2 : Trigonometry
  Trigonometric Function3 : Trigonometry  Operator=tanh
  Trigonometric Function4 : Trigonometry  Operator=tanh
  kx : Gain  Gain=kx/lx  SaturateOnIntegerOverflow=on  OutDataTypeStr=Inherit: Same as input  ParamDataTypeStr=Inherit: Same as input
  ky : Gain  Gain=ky/ly  SaturateOnIntegerOverflow=on  OutDataTypeStr=Inherit: Same as input  ParamDataTypeStr=Inherit: Same as input
  lx : Gain  Gain=lx  SaturateOnIntegerOverflow=on  OutDataTypeStr=Inherit: Same as input  ParamDataTypeStr=Inherit: Same as input
  ly : Gain  Gain=ly  SaturateOnIntegerOverflow=on  OutDataTypeStr=Inherit: Same as input  ParamDataTypeStr=Inherit: Same as input
  psi1 : InportShadow  Port=3
  vel limit : Saturate  UpperLimit=Vmax  LowerLimit=-0.4*Vmax
  w limit : Saturate  UpperLimit=Wmax  LowerLimit=-Wmax
  x1 : InportShadow
  xd1 : InportShadow  Port=4
  y1 : InportShadow  Port=2
  yd1 : InportShadow  Port=5
  ud : Outport
  wd : Outport  Port=2
  targetdir : Outport  Port=3
  wires:
  kx/1 -> Trigonometric Function3/1
  ky/1 -> Trigonometric Function/1
  Trigonometric Function1/1 -> Product3/2, Product/1
  Sum/1 -> kx/1
  y/1 -> Sum2/1
  Sum4/1 -> Product1/1, Product3/1
  Trigonometric Function2/1 -> Product2/2, Product1/2
  Sum3/1 -> vel limit/1
  dxd/1 -> Sum1/2
  dyd/1 -> Sum4/2
  ly/1 -> Sum4/1
  Trigonometric Function/1 -> ly/1
  lx/1 -> Sum1/1
  Trigonometric Function3/1 -> lx/1
  yd/1 -> Sum2/2
  xd/1 -> Sum/2
  x/1 -> Sum/1
  psi/1 -> Trigonometric Function2/1, Trigonometric Function1/1
  Sum1/1 -> Product2/1, Product/2
  Sum2/1 -> ky/1
  Product/1 -> Sum3/1
  Product1/1 -> Sum3/2
  Product3/1 -> Sum5/1
  Product2/1 -> Sum5/2
  Sum5/1 -> 1/a/1
  Trigonometric Function4/1 -> Sum6/1
  1/a/1 -> Trigonometric Function4/1
  vel limit/1 -> ud/1
  w limit/1 -> wd/1
  1/a2/1 -> w limit/1
  Sum6/1 -> 1/a2/1
  psid/1 -> MATLAB Function/2(psid)
  psi1/1 -> MATLAB Function/1(psi)
  x1/1 -> MATLAB Function/3(x)
  xd1/1 -> MATLAB Function/4(xd)
  y1/1 -> MATLAB Function/5(y)
  yd1/1 -> MATLAB Function/6(yd)
  MATLAB Function/1(dw) -> Sum6/2
  MATLAB Function/2(targetdir) -> targetdir/1

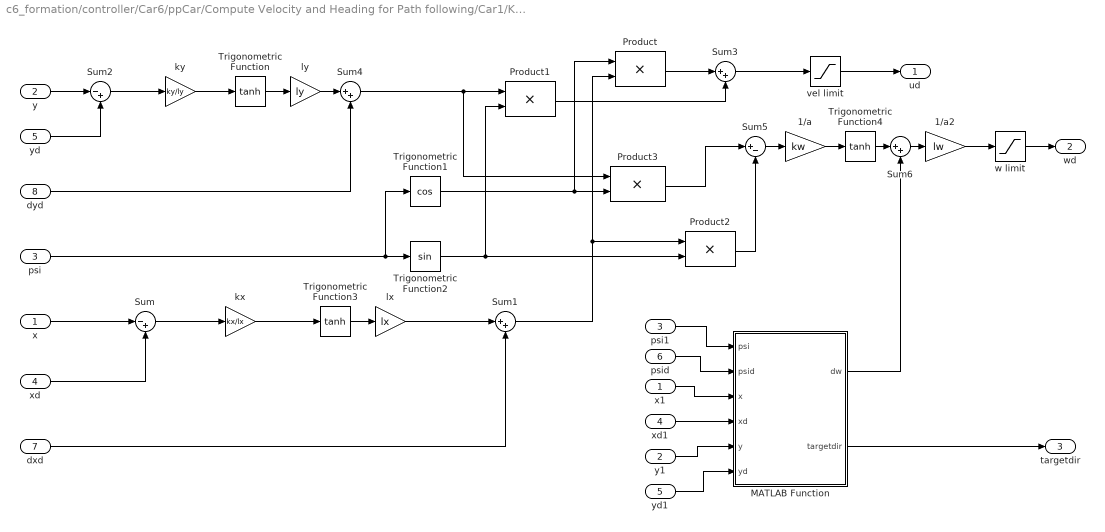
== system c6_formation/controller/Car6/ppCar/Compute Velocity and Heading for Path following/Car1/Kinematicc Controller ==
  x : Inport
  y : Inport  Port=2
  psi : Inport  Port=3
  xd : Inport  Port=4
  yd : Inport  Port=5
  psid : Inport  Port=6
  dxd : Inport  Port=7
  dyd : Inport  Port=8
  1/a : Gain  Gain=kw  SaturateOnIntegerOverflow=on  OutDataTypeStr=Inherit: Same as input  ParamDataTypeStr=Inherit: Same as input
  1/a2 : Gain  Gain=lw  SaturateOnIntegerOverflow=on  OutDataTypeStr=Inherit: Same as input  ParamDataTypeStr=Inherit: Same as input
  MATLAB Function : MATLAB Function  TreatAsAtomicUnit=on
  Product{,1..3} (4 alike) : Product  SaturateOnIntegerOverflow=on  OutDataTypeStr=Inherit: Same as first input
  Sum : Sum  Inputs=|-+  SaturateOnIntegerOverflow=on
  Sum{1,3..4,6} (4 alike) : Sum  Inputs=|++  SaturateOnIntegerOverflow=on
  Sum2 : Sum  Inputs=|-+  SaturateOnIntegerOverflow=on
  Sum5 : Sum  Inputs=|+-  SaturateOnIntegerOverflow=on
  Trigonometric Function : Trigonometry  Operator=tanh
  Trigonometric Function1 : Trigonometry  Operator=cos
  Trigonometric Function2 : Trigonometry
  Trigonometric Function3 : Trigonometry  Operator=tanh
  Trigonometric Function4 : Trigonometry  Operator=tanh
  kx : Gain  Gain=kx/lx  SaturateOnIntegerOverflow=on  OutDataTypeStr=Inherit: Same as input  ParamDataTypeStr=Inherit: Same as input
  ky : Gain  Gain=ky/ly  SaturateOnIntegerOverflow=on  OutDataTypeStr=Inherit: Same as input  ParamDataTypeStr=Inherit: Same as input
  lx : Gain  Gain=lx  SaturateOnIntegerOverflow=on  OutDataTypeStr=Inherit: Same as input  ParamDataTypeStr=Inherit: Same as input
  ly : Gain  Gain=ly  SaturateOnIntegerOverflow=on  OutDataTypeStr=Inherit: Same as input  ParamDataTypeStr=Inherit: Same as input
  psi1 : InportShadow  Port=3
  vel limit : Saturate  UpperLimit=Vmax  LowerLimit=-0.4*Vmax
  w limit : Saturate  UpperLimit=Wmax  LowerLimit=-Wmax
  x1 : InportShadow
  xd1 : InportShadow  Port=4
  y1 : InportShadow  Port=2
  yd1 : InportShadow  Port=5
  ud : Outport
  wd : Outport  Port=2
  targetdir : Outport  Port=3
  wires:
  MATLAB Function/2(targetdir) -> targetdir/1
  MATLAB Function/1(dw) -> Sum6/2
  yd1/1 -> MATLAB Function/6(yd)
  y1/1 -> MATLAB Function/5(y)
  xd1/1 -> MATLAB Function/4(xd)
  x1/1 -> MATLAB Function/3(x)
  psi1/1 -> MATLAB Function/1(psi)
  psid/1 -> MATLAB Function/2(psid)
  Sum6/1 -> 1/a2/1
  1/a2/1 -> w limit/1
  w limit/1 -> wd/1
  vel limit/1 -> ud/1
  1/a/1 -> Trigonometric Function4/1
  Trigonometric Function4/1 -> Sum6/1
  Sum5/1 -> 1/a/1
  Product2/1 -> Sum5/2
  Product3/1 -> Sum5/1
  Product1/1 -> Sum3/2
  Product/1 -> Sum3/1
  Sum2/1 -> ky/1
  Sum1/1 -> Product/2, Product2/1
  psi/1 -> Trigonometric Function1/1, Trigonometric Function2/1
  x/1 -> Sum/1
  xd/1 -> Sum/2
  yd/1 -> Sum2/2
  Trigonometric Function3/1 -> lx/1
  lx/1 -> Sum1/1
  Trigonometric Function/1 -> ly/1
  ly/1 -> Sum4/1
  dyd/1 -> Sum4/2
  dxd/1 -> Sum1/2
  Sum3/1 -> vel limit/1
  Trigonometric Function2/1 -> Product1/2, Product2/2
  Sum4/1 -> Product3/1, Product1/1
  y/1 -> Sum2/1
  Sum/1 -> kx/1
  Trigonometric Function1/1 -> Product/1, Product3/2
  ky/1 -> Trigonometric Function/1
  kx/1 -> Trigonometric Function3/1

== matlab function c6_formation/controller/Car2/ppCar/Adjust Velocities to Avoid Obstacles/Path Following/Compute Angular Velocity ==
  data: steeringDir input; w output; wMax input
function w = exampleHelperComputeAngularVelocity(steeringDir, wMax)
%EXAMPLEHELPERCOMPUTEANGULARVELOCITY Compute angular velocity
%   W = exampleHelperComputeAngularVelocity(STEERINGDIR)
%   returns the angular velocity W for a differential drive robot in radians
%   per second for a given steering direction STEERINGDIR in the robot's
%   coordinate frame in radians.
%
%   W = exampleHelperComputeAngularVelocity(STEERINGDIR, WMAX)
%   returns the angular velocity W for a differential drive robot in radians
%   per second for a given steering direction STEERINGDIR in the robot's
%   coordinate frame in radians and maximum angular velocity WMAX in
%   radians per second. The output angular velocity is saturated based on
%   the WMAX.
%
%   Example:
%       
%       w = exampleHelperComputeAngularVelocity(0.2, 1);

% Copyright 2015 The MathWorks, Inc.

%#codegen
%#ok<*EMCA>

% Allow variable input arguments
if nargin == 1   
    wMax = inf;
end

validateattributes(steeringDir, {'double'},{'real'},...
    'exampleHelperComputeAngularVelocity', 'STEERINGDIR', 1);
validateattributes(wMax, {'double'},{'real', 'positive'},...
    'exampleHelperComputeAngularVelocity', 'WMAX', 2);

% Computing in robot's coordinate frame
curPose = [0 0 0];

% The following computation is similar to robotics.PurePursuit
lookaheadPoint = [cos(steeringDir), sin(steeringDir)];
slope = atan2((lookaheadPoint(2) - curPose(2)), ...
    (lookaheadPoint(1) - curPose(1)));
alpha = angdiff(curPose(3), slope);

% Angular velocity command for a differential drive robot is
% equal to the desired curvature to be followed by the robot.

w = (2*sin(alpha));

% Pick a constant rotation when robot is facing in the opposite
% direction of the path
if abs(abs(alpha) - pi) < 1e-12
    w = sign(w)*1;
end

if abs(w) > wMax
    w = sign(w)*wMax;
end

end

== matlab function c6_formation/controller/Car2/ppCar/Compute Velocity and Heading for Path following/Car1/Kinematicc Controller/MATLAB Function ==
  data: psi input; dw output; psid input; x input; xd input; y input; yd input; targetdir output
function [dw,targetdir]= fcn(psi,psid,x,xd,y,yd)

if norm([xd-x,yd-y])<0.05    
    targetdir=angdiff(psi,psid);
    dw=tanh(targetdir);
else
    dw=0;
    targetdir=angdiff(psi,atan2(yd-y,xd-x));
end

== matlab function c6_formation/controller/Car3/ppCar/Adjust Velocities to Avoid Obstacles/Path Following/Compute Angular Velocity ==
  data: steeringDir input; w output; wMax input
function w = exampleHelperComputeAngularVelocity(steeringDir, wMax)
%EXAMPLEHELPERCOMPUTEANGULARVELOCITY Compute angular velocity
%   W = exampleHelperComputeAngularVelocity(STEERINGDIR)
%   returns the angular velocity W for a differential drive robot in radians
%   per second for a given steering direction STEERINGDIR in the robot's
%   coordinate frame in radians.
%
%   W = exampleHelperComputeAngularVelocity(STEERINGDIR, WMAX)
%   returns the angular velocity W for a differential drive robot in radians
%   per second for a given steering direction STEERINGDIR in the robot's
%   coordinate frame in radians and maximum angular velocity WMAX in
%   radians per second. The output angular velocity is saturated based on
%   the WMAX.
%
%   Example:
%       
%       w = exampleHelperComputeAngularVelocity(0.2, 1);

% Copyright 2015 The MathWorks, Inc.

%#codegen
%#ok<*EMCA>

% Allow variable input arguments
if nargin == 1   
    wMax = inf;
end

validateattributes(steeringDir, {'double'},{'real'},...
    'exampleHelperComputeAngularVelocity', 'STEERINGDIR', 1);
validateattributes(wMax, {'double'},{'real', 'positive'},...
    'exampleHelperComputeAngularVelocity', 'WMAX', 2);

% Computing in robot's coordinate frame
curPose = [0 0 0];

% The following computation is similar to robotics.PurePursuit
lookaheadPoint = [cos(steeringDir), sin(steeringDir)];
slope = atan2((lookaheadPoint(2) - curPose(2)), ...
    (lookaheadPoint(1) - curPose(1)));
alpha = angdiff(curPose(3), slope);

% Angular velocity command for a differential drive robot is
% equal to the desired curvature to be followed by the robot.

w = (2*sin(alpha));

% Pick a constant rotation when robot is facing in the opposite
% direction of the path
if abs(abs(alpha) - pi) < 1e-12
    w = sign(w)*1;
end

if abs(w) > wMax
    w = sign(w)*wMax;
end

end

== matlab function c6_formation/controller/Car3/ppCar/Compute Velocity and Heading for Path following/Car1/Kinematicc Controller/MATLAB Function ==
  data: psi input; dw output; psid input; x input; xd input; y input; yd input; targetdir output
function [dw,targetdir]= fcn(psi,psid,x,xd,y,yd)

if norm([xd-x,yd-y])<0.05    
    targetdir=angdiff(psi,psid);
    dw=tanh(targetdir);
else
    dw=0;
    targetdir=angdiff(psi,atan2(yd-y,xd-x));
end

== matlab function c6_formation/Subsystem/Car Pose Listener1/Subsystem/sensor2vCar ==
  data: x_init output; y_init output; yaw_init output; flag output; poseNew input; poseMsg input
function [x_init,y_init,yaw_init,flag] = sensor2vCar(poseNew, poseMsg)
persistent x0 y0 yaw0 yaw1 x0_init y0_init yaw0_init fStart
if isempty(x0)
    x0=-10; y0=-10; yaw0=0; yaw1=0;   
    x0_init=-10;y0_init=-10;yaw0_init=0;
    fStart=0;
end
if poseNew
    if x0==poseMsg.Pose.Pose.Position.X&&y0==poseMsg.Pose.Pose.Position.Y
        flag=1;
    else
        x0=poseMsg.Pose.Pose.Position.X;
        y0=poseMsg.Pose.Pose.Position.Y;   
        %yaw2=atan2(2*(poseMsg.Pose.Pose.Orientation.Z*poseMsg.Pose.Pose.Orientation.W),1-2*(poseMsg.Pose.Pose.Orientation.Z^2)); 
        eul=quat2eul([poseMsg.Pose.Pose.Orientation.W,poseMsg.Pose.Pose.Orientation.X,poseMsg.Pose.Pose.Orientation.Y,poseMsg.Pose.Pose.Orientation.Z]);
        yaw2=eul(1);
        %对前后角度差使用积分，恢复yaw的连续性
        yaw0=yaw0+angdiff(yaw1,yaw2);
        yaw1=yaw2;
        flag=0;        
        x0_init=x0;
        y0_init=y0;
        yaw0_init=yaw0;
        fStart=1;
    end 
else
    if fStart
        flag=1;
    else
        flag=0;
    end
end

x_init=x0_init;y_init=y0_init;yaw_init=yaw0_init;

== matlab function c6_formation/controller/Car4/ppCar/Adjust Velocities to Avoid Obstacles/Path Following/Compute Angular Velocity ==
  data: steeringDir input; w output; wMax input
function w = exampleHelperComputeAngularVelocity(steeringDir, wMax)
%EXAMPLEHELPERCOMPUTEANGULARVELOCITY Compute angular velocity
%   W = exampleHelperComputeAngularVelocity(STEERINGDIR)
%   returns the angular velocity W for a differential drive robot in radians
%   per second for a given steering direction STEERINGDIR in the robot's
%   coordinate frame in radians.
%
%   W = exampleHelperComputeAngularVelocity(STEERINGDIR, WMAX)
%   returns the angular velocity W for a differential drive robot in radians
%   per second for a given steering direction STEERINGDIR in the robot's
%   coordinate frame in radians and maximum angular velocity WMAX in
%   radians per second. The output angular velocity is saturated based on
%   the WMAX.
%
%   Example:
%       
%       w = exampleHelperComputeAngularVelocity(0.2, 1);

% Copyright 2015 The MathWorks, Inc.

%#codegen
%#ok<*EMCA>

% Allow variable input arguments
if nargin == 1   
    wMax = inf;
end

validateattributes(steeringDir, {'double'},{'real'},...
    'exampleHelperComputeAngularVelocity', 'STEERINGDIR', 1);
validateattributes(wMax, {'double'},{'real', 'positive'},...
    'exampleHelperComputeAngularVelocity', 'WMAX', 2);

% Computing in robot's coordinate frame
curPose = [0 0 0];

% The following computation is similar to robotics.PurePursuit
lookaheadPoint = [cos(steeringDir), sin(steeringDir)];
slope = atan2((lookaheadPoint(2) - curPose(2)), ...
    (lookaheadPoint(1) - curPose(1)));
alpha = angdiff(curPose(3), slope);

% Angular velocity command for a differential drive robot is
% equal to the desired curvature to be followed by the robot.

w = (2*sin(alpha));

% Pick a constant rotation when robot is facing in the opposite
% direction of the path
if abs(abs(alpha) - pi) < 1e-12
    w = sign(w)*1;
end

if abs(w) > wMax
    w = sign(w)*wMax;
end

end

== matlab function c6_formation/controller/Car4/ppCar/Compute Velocity and Heading for Path following/Car1/Kinematicc Controller/MATLAB Function ==
  data: psi input; dw output; psid input; x input; xd input; y input; yd input; targetdir output
function [dw,targetdir]= fcn(psi,psid,x,xd,y,yd)

if norm([xd-x,yd-y])<0.05    
    targetdir=angdiff(psi,psid);
    dw=tanh(targetdir);
else
    dw=0;
    targetdir=angdiff(psi,atan2(yd-y,xd-x));
end

== matlab function c6_formation/Subsystem/Car Pose Listener/Subsystem/sensor2vCar4 ==
  data: V output; W output; VW_New input; VW_Msg input
function [V,W] = sensor2vCar(VW_New, VW_Msg)
persistent v0 w0
if isempty(v0)
    v0=0; 
    w0=0;    
end
if VW_New
    v0=VW_Msg.Linear.X;
    w0=VW_Msg.Angular.Z;
end

V=v0;
W=-w0;

== matlab function c6_formation/controller/Car5/ppCar/Adjust Velocities to Avoid Obstacles/Path Following/Compute Angular Velocity ==
  data: steeringDir input; w output; wMax input
function w = exampleHelperComputeAngularVelocity(steeringDir, wMax)
%EXAMPLEHELPERCOMPUTEANGULARVELOCITY Compute angular velocity
%   W = exampleHelperComputeAngularVelocity(STEERINGDIR)
%   returns the angular velocity W for a differential drive robot in radians
%   per second for a given steering direction STEERINGDIR in the robot's
%   coordinate frame in radians.
%
%   W = exampleHelperComputeAngularVelocity(STEERINGDIR, WMAX)
%   returns the angular velocity W for a differential drive robot in radians
%   per second for a given steering direction STEERINGDIR in the robot's
%   coordinate frame in radians and maximum angular velocity WMAX in
%   radians per second. The output angular velocity is saturated based on
%   the WMAX.
%
%   Example:
%       
%       w = exampleHelperComputeAngularVelocity(0.2, 1);

% Copyright 2015 The MathWorks, Inc.

%#codegen
%#ok<*EMCA>

% Allow variable input arguments
if nargin == 1   
    wMax = inf;
end

validateattributes(steeringDir, {'double'},{'real'},...
    'exampleHelperComputeAngularVelocity', 'STEERINGDIR', 1);
validateattributes(wMax, {'double'},{'real', 'positive'},...
    'exampleHelperComputeAngularVelocity', 'WMAX', 2);

% Computing in robot's coordinate frame
curPose = [0 0 0];

% The following computation is similar to robotics.PurePursuit
lookaheadPoint = [cos(steeringDir), sin(steeringDir)];
slope = atan2((lookaheadPoint(2) - curPose(2)), ...
    (lookaheadPoint(1) - curPose(1)));
alpha = angdiff(curPose(3), slope);

% Angular velocity command for a differential drive robot is
% equal to the desired curvature to be followed by the robot.

w = (2*sin(alpha));

% Pick a constant rotation when robot is facing in the opposite
% direction of the path
if abs(abs(alpha) - pi) < 1e-12
    w = sign(w)*1;
end

if abs(w) > wMax
    w = sign(w)*wMax;
end

end

== matlab function c6_formation/controller/Car5/ppCar/Compute Velocity and Heading for Path following/Car1/Kinematicc Controller/MATLAB Function ==
  data: psi input; dw output; psid input; x input; xd input; y input; yd input; targetdir output
function [dw,targetdir]= fcn(psi,psid,x,xd,y,yd)

if norm([xd-x,yd-y])<0.05    
    targetdir=angdiff(psi,psid);
    dw=tanh(targetdir);
else
    dw=0;
    targetdir=angdiff(psi,atan2(yd-y,xd-x));
end

== matlab function c6_formation/controller/Car6/ppCar/Adjust Velocities to Avoid Obstacles/Path Following/Compute Angular Velocity ==
  data: steeringDir input; w output; wMax input
function w = exampleHelperComputeAngularVelocity(steeringDir, wMax)
%EXAMPLEHELPERCOMPUTEANGULARVELOCITY Compute angular velocity
%   W = exampleHelperComputeAngularVelocity(STEERINGDIR)
%   returns the angular velocity W for a differential drive robot in radians
%   per second for a given steering direction STEERINGDIR in the robot's
%   coordinate frame in radians.
%
%   W = exampleHelperComputeAngularVelocity(STEERINGDIR, WMAX)
%   returns the angular velocity W for a differential drive robot in radians
%   per second for a given steering direction STEERINGDIR in the robot's
%   coordinate frame in radians and maximum angular velocity WMAX in
%   radians per second. The output angular velocity is saturated based on
%   the WMAX.
%
%   Example:
%       
%       w = exampleHelperComputeAngularVelocity(0.2, 1);

% Copyright 2015 The MathWorks, Inc.

%#codegen
%#ok<*EMCA>

% Allow variable input arguments
if nargin == 1   
    wMax = inf;
end

validateattributes(steeringDir, {'double'},{'real'},...
    'exampleHelperComputeAngularVelocity', 'STEERINGDIR', 1);
validateattributes(wMax, {'double'},{'real', 'positive'},...
    'exampleHelperComputeAngularVelocity', 'WMAX', 2);

% Computing in robot's coordinate frame
curPose = [0 0 0];

% The following computation is similar to robotics.PurePursuit
lookaheadPoint = [cos(steeringDir), sin(steeringDir)];
slope = atan2((lookaheadPoint(2) - curPose(2)), ...
    (lookaheadPoint(1) - curPose(1)));
alpha = angdiff(curPose(3), slope);

% Angular velocity command for a differential drive robot is
% equal to the desired curvature to be followed by the robot.

w = (2*sin(alpha));

% Pick a constant rotation when robot is facing in the opposite
% direction of the path
if abs(abs(alpha) - pi) < 1e-12
    w = sign(w)*1;
end

if abs(w) > wMax
    w = sign(w)*wMax;
end

end

== matlab function c6_formation/controller/Car6/ppCar/Compute Velocity and Heading for Path following/Car1/Kinematicc Controller/MATLAB Function ==
  data: psi input; dw output; psid input; x input; xd input; y input; yd input; targetdir output
function [dw,targetdir]= fcn(psi,psid,x,xd,y,yd)

if norm([xd-x,yd-y])<0.05    
    targetdir=angdiff(psi,psid);
    dw=tanh(targetdir);
else
    dw=0;
    targetdir=angdiff(psi,atan2(yd-y,xd-x));
end

== matlab function c6_formation/controller/Car1/ppCar/Adjust Velocities to Avoid Obstacles/Path Following/Compute Angular Velocity ==
  data: steeringDir input; w output; wMax input
function w = exampleHelperComputeAngularVelocity(steeringDir, wMax)
%EXAMPLEHELPERCOMPUTEANGULARVELOCITY Compute angular velocity
%   W = exampleHelperComputeAngularVelocity(STEERINGDIR)
%   returns the angular velocity W for a differential drive robot in radians
%   per second for a given steering direction STEERINGDIR in the robot's
%   coordinate frame in radians.
%
%   W = exampleHelperComputeAngularVelocity(STEERINGDIR, WMAX)
%   returns the angular velocity W for a differential drive robot in radians
%   per second for a given steering direction STEERINGDIR in the robot's
%   coordinate frame in radians and maximum angular velocity WMAX in
%   radians per second. The output angular velocity is saturated based on
%   the WMAX.
%
%   Example:
%       
%       w = exampleHelperComputeAngularVelocity(0.2, 1);

% Copyright 2015 The MathWorks, Inc.

%#codegen
%#ok<*EMCA>

% Allow variable input arguments
if nargin == 1   
    wMax = inf;
end

validateattributes(steeringDir, {'double'},{'real'},...
    'exampleHelperComputeAngularVelocity', 'STEERINGDIR', 1);
validateattributes(wMax, {'double'},{'real', 'positive'},...
    'exampleHelperComputeAngularVelocity', 'WMAX', 2);

% Computing in robot's coordinate frame
curPose = [0 0 0];

% The following computation is similar to robotics.PurePursuit
lookaheadPoint = [cos(steeringDir), sin(steeringDir)];
slope = atan2((lookaheadPoint(2) - curPose(2)), ...
    (lookaheadPoint(1) - curPose(1)));
alpha = angdiff(curPose(3), slope);

% Angular velocity command for a differential drive robot is
% equal to the desired curvature to be followed by the robot.

w = (2*sin(alpha));

% Pick a constant rotation when robot is facing in the opposite
% direction of the path
if abs(abs(alpha) - pi) < 1e-12
    w = sign(w)*1;
end

if abs(w) > wMax
    w = sign(w)*wMax;
end

end

== matlab function c6_formation/Subsystem/Car Pose Listener3/Subsystem/sensor2vCar ==
  data: x_init output; y_init output; yaw_init output; flag output; poseNew input; poseMsg input
function [x_init,y_init,yaw_init,flag] = sensor2vCar(poseNew, poseMsg)
persistent x0 y0 yaw0 yaw1 x0_init y0_init yaw0_init fStart
if isempty(x0)
    x0=-10; y0=-10; yaw0=0; yaw1=0;   
    x0_init=-10;y0_init=-10;yaw0_init=0;
    fStart=0;
end
if poseNew
    if x0==poseMsg.Pose.Pose.Position.X&&y0==poseMsg.Pose.Pose.Position.Y
        flag=1;
    else
        x0=poseMsg.Pose.Pose.Position.X;
        y0=poseMsg.Pose.Pose.Position.Y;   
        %yaw2=atan2(2*(poseMsg.Pose.Pose.Orientation.Z*poseMsg.Pose.Pose.Orientation.W),1-2*(poseMsg.Pose.Pose.Orientation.Z^2)); 
        eul=quat2eul([poseMsg.Pose.Pose.Orientation.W,poseMsg.Pose.Pose.Orientation.X,poseMsg.Pose.Pose.Orientation.Y,poseMsg.Pose.Pose.Orientation.Z]);
        yaw2=eul(1);
        %对前后角度差使用积分，恢复yaw的连续性
        yaw0=yaw0+angdiff(yaw1,yaw2);
        yaw1=yaw2;
        flag=0;        
        x0_init=x0;
        y0_init=y0;
        yaw0_init=yaw0;
        fStart=1;
    end 
else
    if fStart
        flag=1;
    else
        flag=0;
    end
end

x_init=x0_init;y_init=y0_init;yaw_init=yaw0_init;
